simulink model "MS_Alternateur"  (R2021b)
settings: Solver=ode45  StartTime=0.0  StopTime=0.050  MaxStep=100e-6  RelTol=1e-6  EnableMultiTasking=on
undefined symbols (not defined in the file): Ts
libraries: spsGroundLib x6, powerlib_extras x3, spsSeriesRLCBranchLib x3, spsVoltageMeasurementLib x3, spsPermanentMagnetSynchronousMachineLib x1, spspowerguiLib x1
settings Model: Creator=obethoux  LastModifiedBy=zhifansong
settings SolverCC: AlgebraicLoopSolver=TrustRegion
settings DataIOCC: LimitDataPoints=on  SaveFormat=Array  SignalLoggingSaveFormat=ModelDataLogs  ReturnWorkspaceOutputs=off
settings OptimizationCC: ExpressionDepthLimit=2147483647  LifeSpan=inf
settings DebuggingCC: UnderspecifiedInitializationDetection=Classic  MergeDetectMultiDrivingBlocksExec=none  SolverPrmCheckMsg=warning  FcnCallInpInsideContextMsg=warning  StateNameClashWarn=warning  SFUnexpectedBacktrackingDiag=warning  SFNoUnconditionalDefaultTransitionDiag=warning  SFExecutionAtInitializationDiag=none  SFMachineParentedDataDiag=warning  ArithmeticOperatorsInVariantConditions=warning
settings HardwareCC: ProdBitPerPointer=32  ProdBitPerSizeT=32  ProdBitPerPtrDiffT=32  ProdLargestAtomicFloat=None  ProdIntDivRoundTo=Undefined  ProdEndianess=Unspecified  ProdWordSize=32  ProdHWDeviceType=32-bit Generic
settings ModelReferenceCC: PropagateSignalLabelsOutOfModel=off
settings SFSimCC: SimUseLocalCustomCode=off  CustomCodeUndefinedFunction=UseInterfaceOnly
settings RTWCC: RTWUseLocalCustomCode=off
settings CodeAppCC: StateflowObjectComments=on
settings GRTTargetCC: TargetLangStandard=C89/C90 (ANSI)  CombineOutputUpdateFcns=off  GRTInterface=on
settings ConfigComp: CovMetricSettings=dw  CovSaveCumulativeToWorkspaceVar=on  CovSaveSingleToWorkspaceVar=on  CovExternalEMLEnable=off
settings SimscapeCC: SimscapeNormalizeSystem=off

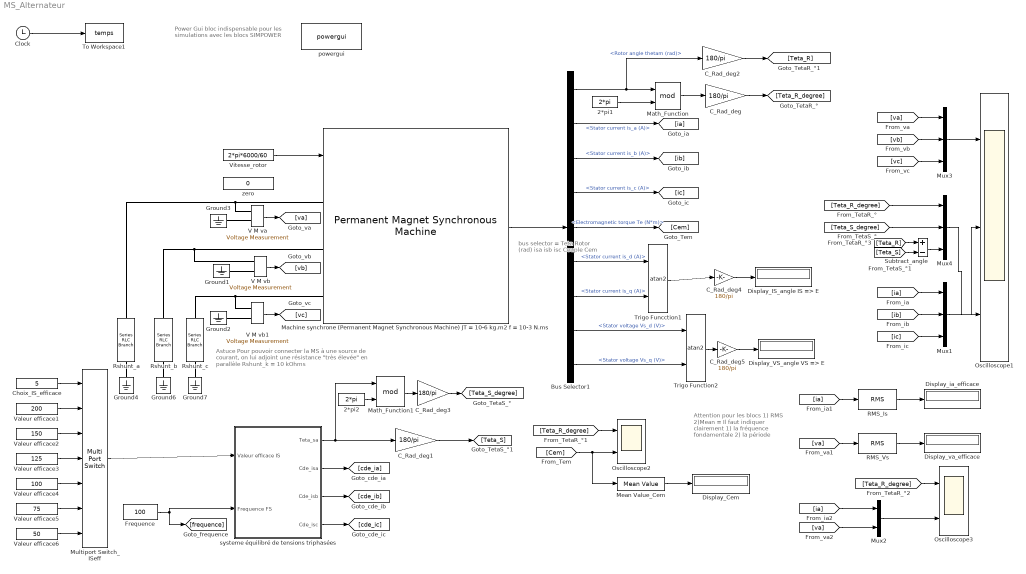
== system MS_Alternateur ==
  note: Power Gui
      | bloc indispensable pour les simulations
      | avec les blocs SIMPOWER
  note: bus selector
      | =
      | Teta Rotor (rad)
      | isa
      | isb
      | isc
      | Couple Cem
  note: Attention pour les blocs
      | 1) RMS
      | 2)Mean
      | =
      | Il faut indiquer clairement
      | 1) la fréquence fondamentale
      | 2) la période
  note: Astuce
      | Pour pouvoir connecter la MS à une source de courant,
      | on lui adjoint une résistance "très élevée" en parallèle
      | Rshunt_k = 10 kOhms
  2*pi1 : Constant  Value=2*pi
  2*pi2 : Constant  Value=2*pi
  Bus Selector1 : BusSelector  OutputSignals=Rotor angle thetam (rad),Stator current is_a (A),Stator current is_b (A),Stator current is_c (A),Electromagnetic torque Te (N*m),Stator current is_d (A),Stator current is_q (A),Stator voltage Vs_d (V),Stator voltage Vs_q (V)
  C_Rad_deg{,1..5} (6 alike) : Gain  Gain=180/pi
  Choix_IS_efficace : Constant  Value=5
  Clock : Clock
  Display_Cem : Display
      settings: Decimation=100
  Display_IS_angle IS => E : Display
      settings: Decimation=100
  Display_VS_angle VS => E : Display
      settings: Decimation=100
  Display_ia_efficace : Display
      settings: Decimation=100
  Display_va_efficace : Display
      settings: Decimation=100
  Frequence : Constant  Value=100
  Ground{1..4,6..7} (6 alike) : spsGroundLib/Ground  LConnTagsString=a
  "Machine synchrone (Permanent Magnet Synchronous Machine) JT = 10-6 kg.m2 f = 10-3 N.ms " : spsPermanentMagnetSynchronousMachineLib/Permanent Magnet Synchronous Machine  NbPhases=3  FluxDistribution=Sinusoidal  RotorType=Round  MechanicalLoad=Speed w  PresetModel=No  ShowDetailedParameters=on  MeasurementBus=off  Resistance=6.75e-3  Inductance=8.5e-3  dqInductances=[8.5e-3,8.5e-3]  La=1.61e-3  MachineConstant=Flux linkage established by magnets (V.s)  Flux=402.5e-3  VoltageCst=73.0054  TorqueCst=0.60375  Flat=120  Mechanical=[1e-6 1e-3 1 0]  PolePairs=1  InitialConditions=[0,0, 0,0]  InitialConditions5ph=[0 0 0 0 0 0]  RefAngle=90 degrees behind phase A axis (modified Park)  IterativeDiscreteModel=Trapezoidal non iterative  TsBlock=-1  TsPowergui=0
  Math_Function : Math  Operator=mod  SignedPower=on  SaturateOnIntegerOverflow=on
  Math_Function1 : Math  Operator=mod  SignedPower=on  SaturateOnIntegerOverflow=on
  Mean Value_Cem : powerlib_extras/Measurements/Mean Value  Period=inv(100)
      settings: SourceProductBaseCode=PS
  Multiport Switch_ISeff : MultiPortSwitch  Inputs=6
  Mux1 : Mux  Inputs=3
  Mux2 : Mux  Inputs=2
  Mux3 : Mux  Inputs=3
  Mux4 : Mux  Inputs=3
  Oscilloscope1 : Scope  NumInputPorts=3
  Oscilloscope2 : Scope  NumInputPorts=2
  Oscilloscope3 : Scope  NumInputPorts=2
  RMS_Is : powerlib_extras/Measurements/RMS  f1=100
      settings: SourceProductBaseCode=PS
  RMS_Vs : powerlib_extras/Measurements/RMS  f1=100
      settings: SourceProductBaseCode=PS
  Rshunt_a : spsSeriesRLCBranchLib/Series RLC Branch  LConnTagsString=__new0  RConnTagsString=__new0  BranchType=R  Resistance=2  Inductance=1e-3  SetiL0=off  InitialCurrent=0  Capacitance=1e-6  Setx0=off  InitialVoltage=0  Measurements=Branch voltage
  Rshunt_b : spsSeriesRLCBranchLib/Series RLC Branch  LConnTagsString=__new0  RConnTagsString=__new0  BranchType=R  Resistance=2  Inductance=1e-3  SetiL0=off  InitialCurrent=0  Capacitance=1e-6  Setx0=off  InitialVoltage=0  Measurements=Branch voltage
  Rshunt_c : spsSeriesRLCBranchLib/Series RLC Branch  LConnTagsString=__new0  RConnTagsString=__new0  BranchType=R  Resistance=2  Inductance=1e-3  SetiL0=off  InitialCurrent=0  Capacitance=1e-6  Setx0=off  InitialVoltage=0  Measurements=Branch voltage
  Subtract_angle : Sum  Inputs=+-
  To Workspace1 : ToWorkspace  VariableName=temps  SampleTime=-1
  Trigo Funcction1 : Trigonometry  Operator=atan2
  Trigo Function2 : Trigonometry  Operator=atan2
  V M va : spsVoltageMeasurementLib/Voltage Measurement  PhasorSimulation=off  OutputType=Complex  PSBequivalent=0
  V M vb : spsVoltageMeasurementLib/Voltage Measurement  PhasorSimulation=off  OutputType=Complex  PSBequivalent=0
  V M vb1 : spsVoltageMeasurementLib/Voltage Measurement  PhasorSimulation=off  OutputType=Complex  PSBequivalent=0
  Valeur efficace1 : Constant  Value=200
  Valeur efficace2 : Constant  Value=150
  Valeur efficace3 : Constant  Value=125
  Valeur efficace4 : Constant  Value=100
  Valeur efficace5 : Constant  Value=75
  Valeur efficace6 : Constant  Value=50
  Vitesse_rotor : Constant  Value=2*pi*6000/60
  powergui : spspowerguiLib/powergui  Priority=2  SimulationMode=Continuous  SampleTime=Ts  frequency=60  Iterations=50  frequencyindice=0  Pbase=100e6  ErrMax=1e-4  UnitsV=kV  UnitsW=MW  buscounter=0  FunctionMessages=off  echomessages=off  EnableUseOfTLC=off  CurrentSourceSwitches=off  DisableSnubberDevices=off  DisableRonSwitches=off  DisableVfSwitches=off  DisplayEquations=off  AutomaticDiscreteSolvers=off  SolverType=Tustin  Interpol=off  ExternalGateDelay=off  methode=off  Ts=0  x0status=blocks  SPID=off  SwTol=0  HookPort=off  NonlinearTolerance=1e-4  nMaxIteration=100  ContinueOnMaxIteration=off  RestoreLinks=warning  ResistiveCurrentMeasurement=off  Frange=[0:2:500]  Ylog=off  Xlog=on  ShowGrid=off  save=off  variable=ZData  structure=0  ZoomFFT=on  StartTime=0.0  cycles=1  DisplayStyle=1  fundamental=60  FreqAxis=off  MaxFrequency=1000  frequencyindicesteady=1  RmsSteady=1  display=off
  systeme équilibré de tensions triphasées : Subsystem
  zero : Constant  Value=0
  wires:
  Clock/1 -> To Workspace1/1
  "Machine synchrone (Permanent Magnet Synchronous Machine) JT = 10-6 kg.m2 f = 10-3 N.ms "/1 -> Bus Selector1/1
  Mux3/1 -> Oscilloscope1/1
  [ia] -> Mux1/1
  [ib] -> Mux1/2
  [ic] -> Mux1/3
  [va] -> Mux3/1
  [vb] -> Mux3/2
  [vc] -> Mux3/3
  Frequence/1 -> systeme équilibré de tensions triphasées/2(Frequence FS), [frequence]
  systeme équilibré de tensions triphasées/2(Cde_isa) -> [cde_ia]
  systeme équilibré de tensions triphasées/3(Cde_isb) -> [cde_ib]
  systeme équilibré de tensions triphasées/4(Cde_isc) -> [cde_ic]
  Bus Selector1/1 -> Math_Function/1, C_Rad_deg2/1  "<Rotor angle thetam (rad)>"
  2*pi1/1 -> Math_Function/2
  Math_Function/1 -> C_Rad_deg/1
  Bus Selector1/2 -> [ia]  "<Stator current is_a (A)>"
  Bus Selector1/3 -> [ib]  "<Stator current is_b (A)>"
  Bus Selector1/4 -> [ic]  "<Stator current is_c (A)>"
  Bus Selector1/5 -> [Cem]  "<Electromagnetic torque Te (N*m)>"
  C_Rad_deg/1 -> [Teta_R_degree]
  [ia] -> RMS_Is/1
  RMS_Is/1 -> Display_ia_efficace/1
  [va] -> RMS_Vs/1
  RMS_Vs/1 -> Display_va_efficace/1
  [Teta_R_degree] -> Oscilloscope2/1
  [Cem] -> Oscilloscope2/2, Mean Value_Cem/1
  Mean Value_Cem/1 -> Display_Cem/1
  V M va/1 -> [va]
  V M vb/1 -> [vb]
  V M vb1/1 -> [vc]
  Multiport Switch_ISeff/1 -> systeme équilibré de tensions triphasées/1(Valeur efficace IS)
  Choix_IS_efficace/1 -> Multiport Switch_ISeff/1
  Mux2/1 -> Oscilloscope3/2
  [Teta_R_degree] -> Oscilloscope3/1
  [va] -> Mux2/2
  [ia] -> Mux2/1
  [Teta_R_degree] -> Mux4/1
  2*pi2/1 -> Math_Function1/2
  systeme équilibré de tensions triphasées/1(Teta_sa) -> C_Rad_deg1/1, Math_Function1/1
  [Teta_R] -> Subtract_angle/1
  C_Rad_deg2/1 -> [Teta_R]
  [Teta_S] -> Subtract_angle/2
  C_Rad_deg1/1 -> [Teta_S]
  Math_Function1/1 -> C_Rad_deg3/1
  C_Rad_deg3/1 -> [Teta_S_degree]
  Valeur efficace6/1 -> Multiport Switch_ISeff/7
  Valeur efficace5/1 -> Multiport Switch_ISeff/6
  Valeur efficace4/1 -> Multiport Switch_ISeff/5
  Valeur efficace3/1 -> Multiport Switch_ISeff/4
  Valeur efficace2/1 -> Multiport Switch_ISeff/3
  Valeur efficace1/1 -> Multiport Switch_ISeff/2
  Trigo Funcction1/1 -> C_Rad_deg4/1
  Trigo Function2/1 -> C_Rad_deg5/1
  C_Rad_deg4/1 -> Display_IS_angle IS => E/1
  C_Rad_deg5/1 -> Display_VS_angle VS => E/1
  Bus Selector1/6 -> Trigo Funcction1/1  "<Stator current is_d (A)>"
  Bus Selector1/7 -> Trigo Funcction1/2  "<Stator current is_q (A)>"
  Bus Selector1/8 -> Trigo Function2/1  "<Stator voltage Vs_d (V)>"
  Bus Selector1/9 -> Trigo Function2/2  "<Stator voltage Vs_q (V)>"
  Vitesse_rotor/1 -> "Machine synchrone (Permanent Magnet Synchronous Machine) JT = 10-6 kg.m2 f = 10-3 N.ms "/1
  Mux4/1 -> Oscilloscope1/3
  Mux1/1 -> Oscilloscope1/2
  [Teta_S_degree] -> Mux4/2
  Subtract_angle/1 -> Mux4/3
  connections:
  Ground3/LConn1 -- V M va/LConn2
  Ground1/LConn1 -- V M vb/LConn2
  V M vb1/LConn2 -- Ground2/LConn1
  "Machine synchrone (Permanent Magnet Synchronous Machine) JT = 10-6 kg.m2 f = 10-3 N.ms "/LConn1 -- Rshunt_a/LConn1 -- V M va/LConn1
  Ground4/LConn1 -- Rshunt_a/RConn1
  Ground6/LConn1 -- Rshunt_b/RConn1
  Ground7/LConn1 -- Rshunt_c/RConn1
  "Machine synchrone (Permanent Magnet Synchronous Machine) JT = 10-6 kg.m2 f = 10-3 N.ms "/LConn2 -- Rshunt_b/LConn1 -- V M vb/LConn1
  "Machine synchrone (Permanent Magnet Synchronous Machine) JT = 10-6 kg.m2 f = 10-3 N.ms "/LConn3 -- Rshunt_c/LConn1 -- V M vb1/LConn1

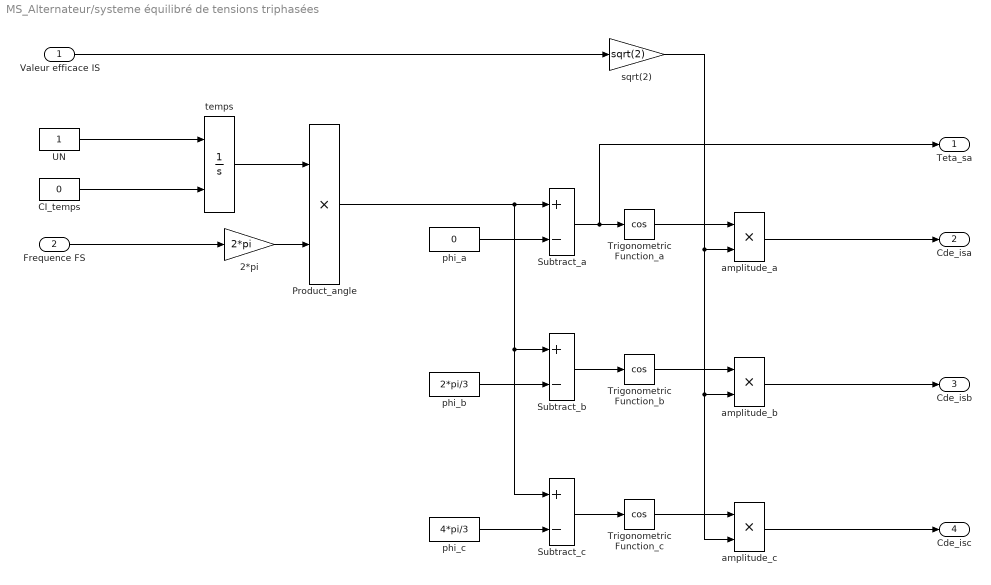
== system MS_Alternateur/systeme équilibré de tensions triphasées ==
  Valeur efficace IS : Inport
  Frequence FS : Inport  Port=2
  2*pi : Gain  Gain=2*pi
  CI_temps : Constant  Value=0
  Product_angle : Product  RndMeth=Zero
  Subtract_a : Sum  Inputs=+-
  Subtract_b : Sum  Inputs=+-
  Subtract_c : Sum  Inputs=+-
  Trigonometric Function_a : Trigonometry  Operator=cos
  Trigonometric Function_b : Trigonometry  Operator=cos
  Trigonometric Function_c : Trigonometry  Operator=cos
  UN : Constant
  amplitude_a : Product  RndMeth=Zero
  amplitude_b : Product  RndMeth=Zero
  amplitude_c : Product  RndMeth=Zero
  phi_a : Constant  Value=0
  phi_b : Constant  Value=2*pi/3
  phi_c : Constant  Value=4*pi/3
  sqrt(2) : Gain  Gain=sqrt(2)
  temps : Integrator  InitialConditionSource=external
  Teta_sa : Outport
  Cde_isa : Outport  Port=2
  Cde_isb : Outport  Port=3
  Cde_isc : Outport  Port=4
  wires:
  CI_temps/1 -> temps/2
  UN/1 -> temps/1
  temps/1 -> Product_angle/1
  2*pi/1 -> Product_angle/2
  phi_a/1 -> Subtract_a/2
  phi_b/1 -> Subtract_b/2
  phi_c/1 -> Subtract_c/2
  Subtract_a/1 -> Trigonometric Function_a/1, Teta_sa/1
  Subtract_b/1 -> Trigonometric Function_b/1
  Subtract_c/1 -> Trigonometric Function_c/1
  Trigonometric Function_a/1 -> amplitude_a/1
  Trigonometric Function_b/1 -> amplitude_b/1
  Trigonometric Function_c/1 -> amplitude_c/1
  sqrt(2)/1 -> amplitude_a/2, amplitude_b/2, amplitude_c/2
  Valeur efficace IS/1 -> sqrt(2)/1
  amplitude_a/1 -> Cde_isa/1
  Frequence FS/1 -> 2*pi/1
  amplitude_b/1 -> Cde_isb/1
  amplitude_c/1 -> Cde_isc/1
  Product_angle/1 -> Subtract_a/1, Subtract_b/1, Subtract_c/1
